simulink model "model"  (R2025b)
settings: Solver=FixedStepAuto  StartTime=0.0  StopTime=50  RelTol=1e-3
values from neighbouring files (symbols this model uses):
  delay = 8    [dane.m]
  dist_ref = 100    [dane.m]
  fs = 100    [dane.m]
  v_lead = 25    [dane.m]
libraries: simulink x3, robotmobilelib x1, robotalgslib x1, simulink_extras x1, slpidlib x1
settings Model: Creator=szymo  LastModifiedBy=Lenovo

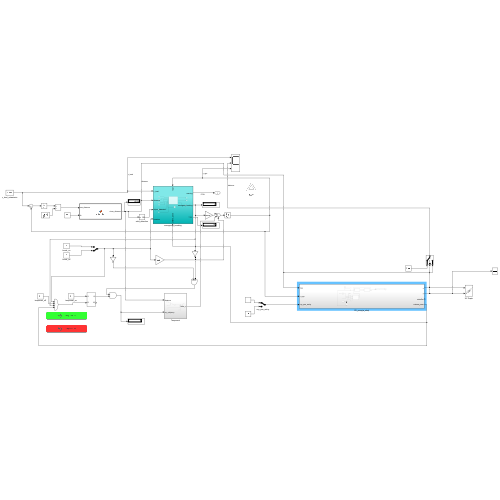
[thumbnail: Simulink's stored preview of the top-level diagram]
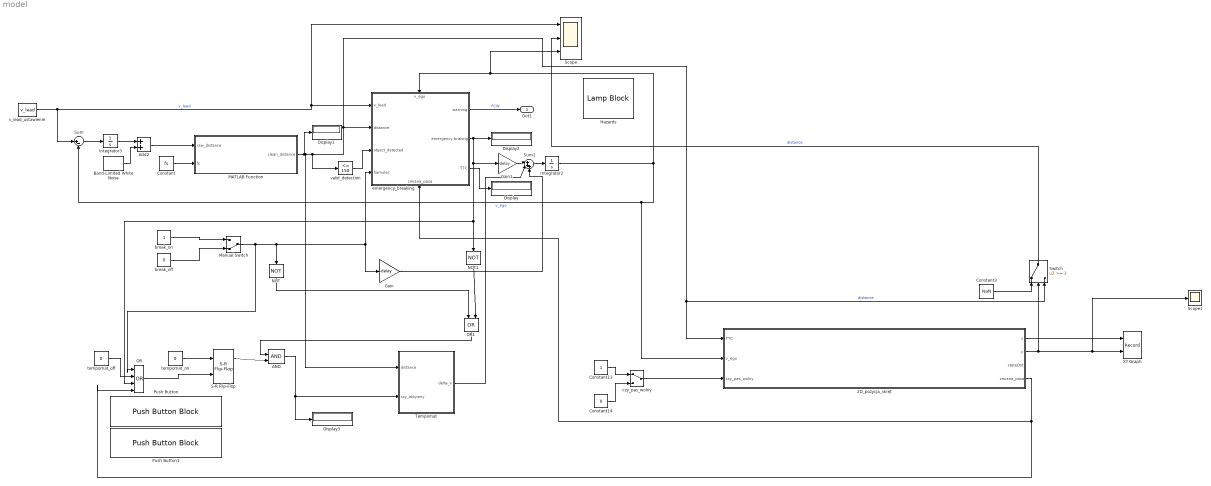
== system model ==
  2D_pozycja_skręt : Subsystem
  AND : Logic  IconShape=distinctive  AllPortsSameDT=off  OutDataTypeStr=boolean
  Add2 : Sum
  Band-Limited White Noise : simulink/Sources/Band-Limited White Noise  Cov=[0.1]  Ts=0.1  seed=[23341]
  Constant : Constant  Value=fs
  Constant13 : Constant
  Constant14 : Constant  Value=0
  Constant3 : Constant  Value=NaN
  Display{,1..3} (4 alike) : Display
  Gain : Gain  Gain=-delay
  Gain1 : Gain  Gain=-delay
  Hazards : LampBlock  LabelPosition=Bottom  DefaultColor=[192.0, 192.0, 192.0]  Icon=Hazards
  Integrator2 : Integrator  InitialCondition=30  LimitOutput=on  LowerSaturationLimit=0
  Integrator3 : Integrator  InitialCondition=200
  MATLAB Function : MATLAB Function  TreatAsAtomicUnit=on
  Manual Switch : ManualSwitch  CurrentSetting=0
  NOT : Logic  Operator=NOT  IconShape=distinctive  AllPortsSameDT=off  OutDataTypeStr=boolean
  NOT1 : Logic  Operator=NOT  IconShape=distinctive  AllPortsSameDT=off  OutDataTypeStr=boolean
  OR : Logic  Operator=OR  Inputs=4  IconShape=distinctive  AllPortsSameDT=off  OutDataTypeStr=boolean
  OR1 : Logic  Operator=OR  IconShape=distinctive  AllPortsSameDT=off  OutDataTypeStr=boolean
  Push Button : PushButtonBlock  ButtonText=Tempomat on  Icon=AdaptiveCruiseControl  IconOnColor=[0.0, 0.39215686274509803, 0.0]  IconOffColor=[0.0, 1.0, 0.0]  OffValue=0.000000
  Push Button1 : PushButtonBlock  ButtonText=Tempomat off  Icon=AdaptiveCruiseControl  IconOnColor=[0.0, 0.39215686274509803, 0.0]  IconOffColor=[0.0, 1.0, 0.0]  OffValue=0.000000
  S-R Flip-Flop : simulink_extras/Flip Flops/S-R Flip-Flop  initial_condition=0
  Scope : Scope  NumInputPorts=3
      settings: ActiveDisplayYMinimum=-56.758446095335444  ActiveDisplayYMaximum=225.73474834867932
  Scope1 : Scope
      settings: ActiveDisplayYMinimum=-0.52982785301315882  ActiveDisplayYMaximum=8.4490965584467048
  Sum : Sum  Inputs=|+-
  Sum2 : Sum  Inputs=|+++
  Switch : Switch  Threshold=3  SaturateOnIntegerOverflow=off  InputSameDT=off
  Tempomat : Subsystem
  XY Graph : Record  NumPorts=2.0  FileSettingsInternal="{\"entries\":[{\"content\":{\"excelSettings\":{\"content\":{},\"type\":\"Streamout.ExcelSettings\"},\"parquetSettings\":{\"content\":{},\"type\":\"Streamout.ParquetSettings\"}},\"type\":\"Streamout.FileSettingStorage\",\"uuid\":\"\"}],\"packageUris\":[\"http:\\/\\/schema.mathworks.com\\/mf0\\/streamout_blocks\\/R2020a\"],\"version\":\"1.0\"}"  FrameSettings=[0, 0]  Layout=[1 1]  SignalsInternal="{\"entries\":[{\"content\":{\"signals\":[{\"content\":{\"blockPath\":[],\"dimensions\":[1],\"domain\":\"\",\"lineColor\":\"#ff13a6\",\"lineWidth\":2,\"plots\":[ 1 ],\"port\":1,\"sid\":[\"\"],\"signalID\":1,\"signalName\":\"2D_pozycja_skręt:1\"},\"type\":\"RecordBlkView.Signal\",\"uuid\":\"\"},{\"content\":{\"blockPath\":[],\"dimensions\":[1],\"domain\":\"\",\"lineColor\":\"#fe330a\",\"lineWidth\":2,\"plots\":[ 1 ],\"port\":2,\"sid\":[\"\"],\"signalID\":2,\"signalName\":\"2D_pozycja_skręt:2\"},\"type\":\"RecordBlkView.Signal\",\"uuid\":\"\"}]},\"type\":\"RecordBlkView.InputSignals\",\"uuid\":\"\"}],\"packageUris\":[\"http:\\/\\/schema.mathworks.com\\/mf0\\/streamout_blocks\\/R2020a\"],\"version\":\"1.0\"}"  VisualizationBindings="{\"xyplotplugin\":{\"info\":[{\"series\":[{\"bindingParametersList\":[{\"parameter\":\"X-Axis\",\"signalID\":1,\"signalName\":\"2D_pozycja_skręt:1\"},{\"parameter\":\"Y-Axis\",\"signalID\":2,\"signalName\":\"2D_pozycja_skręt:2\"}],\"seriesID\":0}],\"subplotID\":1}]}}"  CompatibilityTag=XY
  break_off : Constant  Value=0
  break_on : Constant
  czy_pas_wolny : ManualSwitch
  emergency_breaking : Subsystem
      settings: PortSchema="{\"entries\":[{\"content\":{\"sides\":[{\"content\":{\"connectorIds\":[\"In1\",\"In2\",\"In3\",\"In4\"]},\"type\":\"ConnectorPlacement.EquallySpacedRectSide\",\"uuid\":\"5c278209-309c-454c-9768-cae4674b78a0\"},{\"content\":{\"connectorIds\":[\"Out1\",\"Out2\",\"Out3\"],\"side\":\"RIGHT\"},\"type\":\"ConnectorPlacement.EquallySpacedRectSide\",\"uuid\":\"aa78647b-400e-407b-8285-1c51700bacef\"},{\"content\":{\"connectorIds\":[\"In5\"],\"side\":\"TOP\"},\"type\":\"ConnectorPlacement.EquallySpacedRectSide\",\"uuid\":\"b03ed96f-f297-436b-9e7c-27fd612abd23\"},{\"content\":{\"connectorIds\":[\"In6\"],\"side\":\"BOTTOM\"},\"type\":\"ConnectorPlacement.EquallySpacedRectSide\",\"uuid\":\"e8fbca29-9a5d-4ac8-8236-b91ec1091407\"}]},\"type\":\"ConnectorPlacement.EquallySpacedConnector\",\"uuid\":\"ec3ffc7b-2362-4feb-b307-32101ef81daa\"}],\"packageUris\":[\"http://schema.mathworks.com/mf0/Connector/R2020b\"],\"version\":\"1.0\"}"
  tempomat_off : Constant  Value=0
  tempomat_on : Constant  Value=0  OutDataTypeStr=boolean
  v_lead_ustawienie : Constant  Value=v_lead
  valid_detection : simulink/Logic and Bit Operations/Compare To Constant  relop=<=  const=150  OutDataTypeStr=boolean
  Out1 : Outport
  wires:
  Band-Limited White Noise/1 -> Add2/2
  Add2/1 -> MATLAB Function/1(raw_distance)
  Constant/1 -> MATLAB Function/2(fs)
  v_lead_ustawienie/1 -> Sum/1, Scope/1, emergency_breaking/1(v_lead)  "v_lead"
  Sum/1 -> Integrator3/1
  Integrator3/1 -> Add2/1
  MATLAB Function/1(clean_distance) -> Switch/3, 2D_pozycja_skręt/1(TTC), emergency_breaking/2(distance), valid_detection/1, Tempomat/1(distance), Display1/1  "distance"
  valid_detection/1 -> emergency_breaking/3(object_detected)
  emergency_breaking/1(warning) -> Out1/1  "FCW"
  emergency_breaking/3("TTC ") -> Display/1
  break_on/1 -> Manual Switch/1
  break_off/1 -> Manual Switch/2
  Gain/1 -> Sum2/3
  tempomat_on/1 -> S-R Flip-Flop/1
  OR/1 -> S-R Flip-Flop/2
  tempomat_off/1 -> OR/2
  NOT/1 -> OR1/1
  S-R Flip-Flop/1 -> AND/2
  AND/1 -> Display3/1, Tempomat/2(czy_aktywny)
  emergency_breaking/2(emergency braking) -> NOT1/1, OR/3, Gain1/1, Display2/1
  Manual Switch/1 -> OR/1, NOT/1, emergency_breaking/4(hamulec), Gain/1
  Integrator2/1 -> 2D_pozycja_skręt/2(v_ego), Sum/2, Scope/3, emergency_breaking/5(v_ego)  "v_ego"
  NOT1/1 -> OR1/2
  OR1/1 -> AND/1
  Gain1/1 -> Sum2/1
  Sum2/1 -> Integrator2/1
  Tempomat/1(delta_v) -> Sum2/2
  2D_pozycja_skręt/1(x) -> XY Graph/1
  2D_pozycja_skręt/2(y) -> Switch/2, Scope1/1, XY Graph/2
  2D_pozycja_skręt/4(zmiana_pasa) -> OR/4, emergency_breaking/6(zmiana_pasa)
  Constant3/1 -> Switch/1
  Switch/1 -> Scope/2  "distance"
  czy_pas_wolny/1 -> 2D_pozycja_skręt/3(czy_pas_wolny)
  Constant13/1 -> czy_pas_wolny/1
  Constant14/1 -> czy_pas_wolny/2

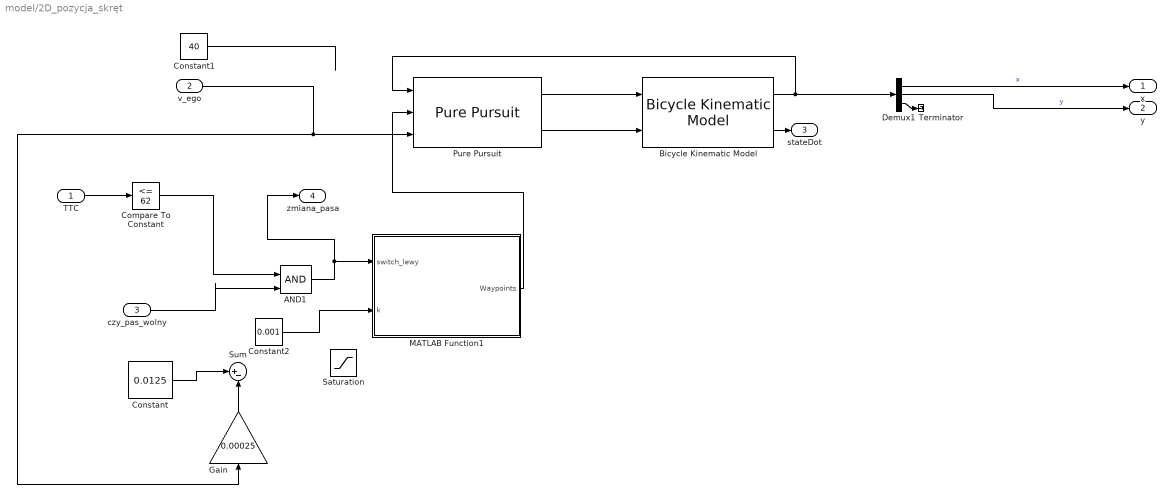
== system model/2D_pozycja_skręt ==
  TTC : Inport
  v_ego : Inport  Port=2
  czy_pas_wolny : Inport  Port=3
  AND1 : Logic  IconShape=distinctive  AllPortsSameDT=off  OutDataTypeStr=boolean
  Bicycle Kinematic Model : robotmobilelib/Bicycle Kinematic Model  VehicleInputs=Vehicle Speed & Heading Angular Velocity  WheelBase=2.7  VehicleSpeedRange=[0.01,100]  MaxSteeringAngle=pi/3  InitialState=[0; 0; 0]  SimulateUsing=Interpreted execution
  Compare To Constant : simulink/Logic and Bit Operations/Compare To Constant  relop=<=  const=62  OutDataTypeStr=boolean
  Constant : Constant  Value=0.0125
  Constant1 : Constant  Value=40
  Constant2 : Constant  Value=0.001
  Demux1 : Demux  Outputs=3
  Gain : Gain  Gain=0.00025
  MATLAB Function1 : MATLAB Function  TreatAsAtomicUnit=on
  Pure Pursuit : robotalgslib/Pure Pursuit  DesiredLinearVelocityPort=on  DesiredLinearVelocity=5  MaxAngularVelocity=1.0  LookaheadDistancePort=off  LookaheadDistance=40  TargetDirPort=off  SimulateUsing=Code generation
      settings: LibrarySourceBlock=navlib/Control Algorithms/Pure Pursuit
  Saturation : Saturate  UpperLimit=0.01  LowerLimit=0.001
  Sum : Sum  Inputs=|+-
  Terminator : Terminator
  x : Outport
  y : Outport  Port=2
  stateDot : Outport  Port=3
  zmiana_pasa : Outport  Port=4
  wires:
  Bicycle Kinematic Model/2 -> stateDot/1
  Demux1/3 -> Terminator/1
  Bicycle Kinematic Model/1 -> Demux1/1, Pure Pursuit/1
  MATLAB Function1/1(Waypoints) -> Pure Pursuit/2
  AND1/1 -> MATLAB Function1/1(switch_lewy), zmiana_pasa/1
  Demux1/1 -> x/1  "x"
  Demux1/2 -> y/1  "y"
  TTC/1 -> Compare To Constant/1
  Pure Pursuit/1 -> Bicycle Kinematic Model/1
  czy_pas_wolny/1 -> AND1/2
  Compare To Constant/1 -> AND1/1
  Constant/1 -> Sum/1
  Gain/1 -> Sum/2
  v_ego/1 -> Pure Pursuit/3, Gain/1
  Pure Pursuit/2 -> Bicycle Kinematic Model/2
  Constant2/1 -> MATLAB Function1/2(k)
  Constant1/1 -> ?

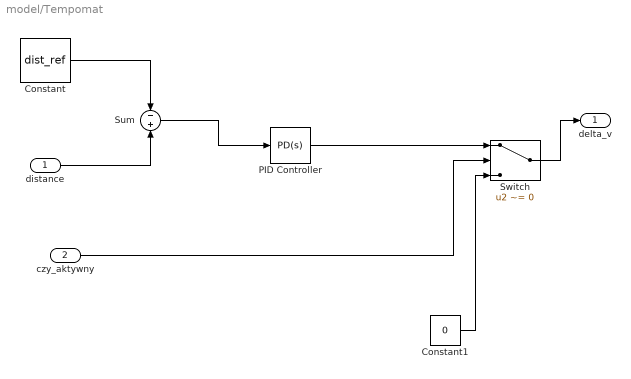
== system model/Tempomat ==
  distance : Inport
  czy_aktywny : Inport  Port=2
  Constant : Constant  Value=dist_ref
  Constant1 : Constant  Value=0
  PID Controller : slpidlib/PID Controller  Controller=PD  Form=Parallel  TimeDomain=Continuous-time  UseExternalTs=off  SampleTime=-1  IntegratorMethod=Forward Euler  FilterMethod=Forward Euler  ControllerParametersSource=internal  P=0.1  I=0  UseKiTs=off  D=0.8  UseExternalDerivativeSource=off  N=10  UseFilter=on  TunerSelectOption=Transfer Function Based (PID Tuner App)  InitialConditionSource=internal  InitialConditionForIntegrator=0  InitialConditionForFilter=0  DifferentiatorICPrevScaledInput=0  ExternalReset=none  TrackingMode=off  Kt=1  LimitOutput=on  SatLimitsSource=internal  UpperSaturationLimit=1.5  LowerSaturationLimit=-2.5  LinearizeAsGain=on  AntiWindupMode=none  Kb=1  LimitIntegrator=off  UpperIntegratorSaturationLimit=inf  LowerIntegratorSaturationLimit=-inf  POutMin=[]  POutMax=[]  IOutMin=[]  IOutMax=[]  DOutMin=[]  DOutMax=[]  NOutMin=[]  NOutMax=[]  SumOutMin=[]  SumOutMax=[]  SaturationOutMin=[]  SaturationOutMax=[]  PParamMin=[]  PParamMax=[]  IParamMin=[]  IParamMax=[]  DParamMin=[]  DParamMax=[]  NParamMin=[]  NParamMax=[]  KbParamMin=[]  KbParamMax=[]  KtParamMin=[]  KtParamMax=[]  KbOutMin=[]  KbOutMax=[]  KtOutMin=[]  KtOutMax=[]  IntegratorOutMin=[]  IntegratorOutMax=[]  FilterOutMin=[]  FilterOutMax=[]  SumI1OutMin=[]  SumI1OutMax=[]  SumI2OutMin=[]  SumI2OutMax=[]  SumI3OutMin=[]  SumI3OutMax=[]  SumI4OutMin=[]  SumI4OutMax=[]  SumDOutMin=[]  SumDOutMax=[]  DifferentiatorOutMin=[]  DifferentiatorOutMax=[]  FilterDiffOutCoefMin=[]  FilterDiffOutCoefMax=[]  ReciprocalOutMin=[]  ReciprocalOutMax=[]  SumDenOutMin=[]  SumDenOutMax=[]  SumNumOutMin=[]  SumNumOutMax=[]  DivideOutMin=[]  DivideOutMax=[]  UdiffTsProdOutMin=[]  UdiffTsProdOutMax=[]  NTsProdOutMin=[]  NTsProdOutMax=[]  UintegralTsProdOutMin=[]  UintegralTsProdOutMax=[]  UngainTsProdOutMin=[]  UngainTsProdOutMax=[]  ClampingZeroOutDataTypeStr=Inherit: Inherit via back propagation  ClampingZeroOutMin=[]  ClampingZeroOutMax=[]  FilterDenConstantOutDataTypeStr=Inherit: Inherit via back propagation  FilterDenConstantOutMin=[]  FilterDenConstantOutMax=[]  PCopyOutDataTypeStr=Inherit: Inherit via back propagation  PCopyOutMin=[]  PCopyOutMax=[]  NCopyOutDataTypeStr=Inherit: Inherit via back propagation  NCopyOutMin=[]  NCopyOutMax=[]  IntegratorContinuousStateAttributes=''  IntegratorStateMustResolveToSignalObject=off  IntegratorRTWStateStorageClass=Auto  FilterContinuousStateAttributes=''  FilterStateMustResolveToSignalObject=off  FilterRTWStateStorageClass=Auto  ParallelPVariant=InternalParameters  IdealPVariant=Disabled  IVariant=Disabled  DVariant=InternalParameters  IntegratorVariant=Disabled  SatVariant=Enabled  AWVariant=Disabled  PCopyVariant=Disabled  TRVariant=Disabled  FdbkBlocksVariant=Forward  IdealPFdbkVariant=Disabled  SatFdbkVariant=Disabled  DerivativeFilterVariant=ContFilter  NVariant=InternalParameters  NCopyVariant=Disabled  FilterICVariant=InternalICsFilter  IntegratorICVariant=Disabled  ExternalResetVariant=Disabled  TRSumVariant=Passthrough  SumFdbkVariant=Disabled  SumVariant=Sum_PD  TsampFilterVariant=InternalTs  TsampNgainVariant=Passthrough  TsampIntegralVariant=Disabled_SignalSpec  ExternalSaturationOutDataTypeStr=Inherit: Same as second input  DerivativeSourceVariant=ErrorSignal  PreIntVariant=InternalPreInt
  Sum : Sum  Inputs=-+
  Switch : Switch  Criteria=u2 ~= 0  SaturateOnIntegerOverflow=off  InputSameDT=off
  delta_v : Outport
  wires:
  czy_aktywny/1 -> Switch/2
  Switch/1 -> delta_v/1
  Constant1/1 -> Switch/3
  PID Controller/1 -> Switch/1
  Sum/1 -> PID Controller/1
  Constant/1 -> Sum/1
  distance/1 -> Sum/2

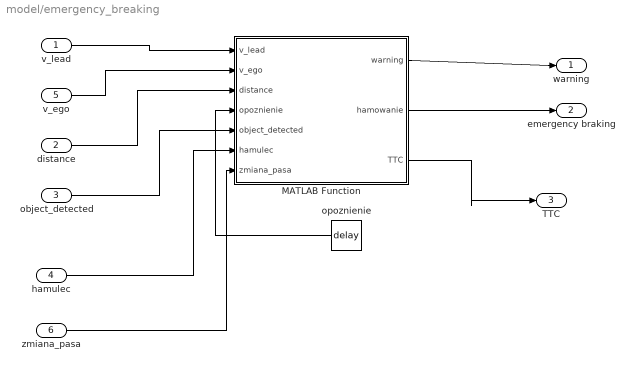
== system model/emergency_breaking ==
  v_lead : Inport
  distance : Inport  Port=2
  object_detected : Inport  Port=3
  hamulec : Inport  Port=4
  v_ego : Inport  Port=5
  zmiana_pasa : Inport  Port=6
  MATLAB Function : MATLAB Function  TreatAsAtomicUnit=on
  opoznienie : Constant  Value=delay
  warning : Outport
  emergency braking : Outport  Port=2
  "TTC " : Outport  Port=3
  wires:
  opoznienie/1 -> MATLAB Function/4(opoznienie)
  distance/1 -> MATLAB Function/3(distance)
  object_detected/1 -> MATLAB Function/5(object_detected)
  MATLAB Function/3(TTC) -> "TTC "/1
  MATLAB Function/1(warning) -> warning/1
  hamulec/1 -> MATLAB Function/6(hamulec)
  v_lead/1 -> MATLAB Function/1(v_lead)
  v_ego/1 -> MATLAB Function/2(v_ego)
  MATLAB Function/2(hamowanie) -> emergency braking/1
  zmiana_pasa/1 -> MATLAB Function/7(zmiana_pasa)

== matlab function model/emergency_breaking/MATLAB Function ==
  data: v_lead input; warning output; hamowanie output; TTC output; v_ego input; distance input; opoznienie input; object_detected input; hamulec input; zmiana_pasa input
function [warning, hamowanie, TTC] = AEB(v_lead, v_ego, distance,  opoznienie, object_detected, hamulec, zmiana_pasa)
    v_wzgl = v_ego - v_lead;  

    if zmiana_pasa == 1
        warning = 0;
        hamowanie = 0;
        TTC = inf;
        return
    end

    if object_detected == 0
        warning =0;
        hamowanie = 0;
        TTC = inf;
        return
    end

    if v_ego <= 0
        hamowanie = 0;
        warning = 0;
        TTC = 999;
        return
    end

    TTC = distance/abs(v_wzgl);
    prog_czasowy = v_wzgl/opoznienie;
    prog_finalny = prog_czasowy + 0.7;

    if TTC<(prog_finalny + 1.0) && TTC >= prog_finalny
        warning = 1;
        hamowanie = 0; 
    elseif TTC < prog_finalny
        warning = 1;  
        if hamulec
            hamowanie=0;
        else
            hamowanie = 1;
        end
    else
        warning = 0;
        hamowanie = 0;
    end
end

== matlab function model/MATLAB Function ==
  settings: updateMethod=DISCRETE
  data: raw_distance input; clean_distance output; fs input
function clean_distance = radar_filter(raw_distance, fs)
    persistent last_dist;
    
    % Inicjalizacja przy pierwszym kroku symulacji
    if isempty(last_dist)
        last_dist = raw_distance;
    end  
    
    % Obliczenie kroku czasu na podstawie częstotliwości próbkowania
    dt = 1 / fs; 
    
    tau = 0.02; 
    
    % Dynamiczne obliczenie wagi dla nowego pomiaru
    alpha = dt / (tau + dt); 
    
    % Filtracja: waga_nowego * nowy_pomiar + waga_starego * stary_pomiar
    clean_distance = alpha * raw_distance + (1 - alpha) * last_dist;
    
    % Zapisanie obecnej wartości na potrzeby kolejnego kroku
    last_dist = clean_distance;
end

== matlab function model/2D_pozycja_skręt/MATLAB Function1 ==
  settings: updateMethod=DISCRETE
  data: switch_lewy input; Waypoints output; k input
%function Waypoints = generuj_trajektorie(switch_lewy, k)
%  function Waypoints = generuj_trajektorie(switch_lewy, k)
%     % Parametry
%     L_symulacji = 5000;  % Całkowity dystans
%     dx = 1.0;            % Rozdzielczość
%     W = 4.0;             % Docelowy lewy pas
% 
%     % Parametr 'k' steruje długością manewru.
%     % Dla k = 0.02 manewr zajmie około 100 metrów.
%     % Jeśli chcesz jeszcze łagodniej, zmniejsz na np. 0.015 lub 0.01             
% 
%     X = (0:dx:L_symulacji)'; 
%     Y = zeros(size(X));
% 
%     if switch_lewy == 1
%         % Zwróć uwagę na potęgę kwadratową (.^2) na zmiennej X.
%         % To ona gwarantuje, że start jest "płaski" i nie szarpie kierownicą.
%         Y = W * (1 - exp(-(k * X).^2));
%     else
%         Y = zeros(size(X));
%     end
% 
%     Waypoints = [X, Y];
% end

function Waypoints = generuj_trajektorie(switch_lewy, k)
    % --- PARAMETRY STAŁE ---
    L_symulacji = 5000;  % Całkowity dystans
    dx = 1.0;            % Rozdzielczość
    W = 4.0;             % Docelowy pas
    
    % Zabezpieczenie na wypadek, gdyby sygnał k z jakiegoś powodu był 0 lub ujemny
    if k <= 0
        k = 0.0001;
    end

    % --- GENEROWANIE WEKTORÓW ---
    X = (0:dx:L_symulacji)'; 
    Y = zeros(size(X));

    if switch_lewy == 1
        % Funkcja ARCUS TANGENS dążąca do asymptoty W=4
        % Oparta na gotowym 'k' podanym na wejście bloku
        X = (0:dx:L_symulacji)';
        Y = (2 * W / pi) * atan((k * X).^2);
    else
        Y = zeros(size(X));
    end

    Waypoints = [X, Y];
end
